simulink model "SECURE_Russia_EU_Ukraine_gas_pipeline"  (Simulink 10.3)
settings: Solver=ode45  StartTime=0.0  StopTime=100  RelTol=1e-3  EnableMultiTasking=on
undefined symbols (not defined in the file): Tab, Tba, Tca, Tcb
settings Model: Creator=Luan Nguyen  LastModifiedBy=fmendoz2  MultithreadedSim=on
settings DataIOCC: LimitDataPoints=on
settings DebuggingCC: IgnoredZcDiagnostic=none  MultiTaskDSMMsg=warning  MultiTaskCondExecSysMsg=none  FcnCallInpInsideContextMsg=error
settings GRTTargetCC: CombineOutputUpdateFcns=on  GRTInterface=off
settings ConfigComp: CovSFcnEnable=off

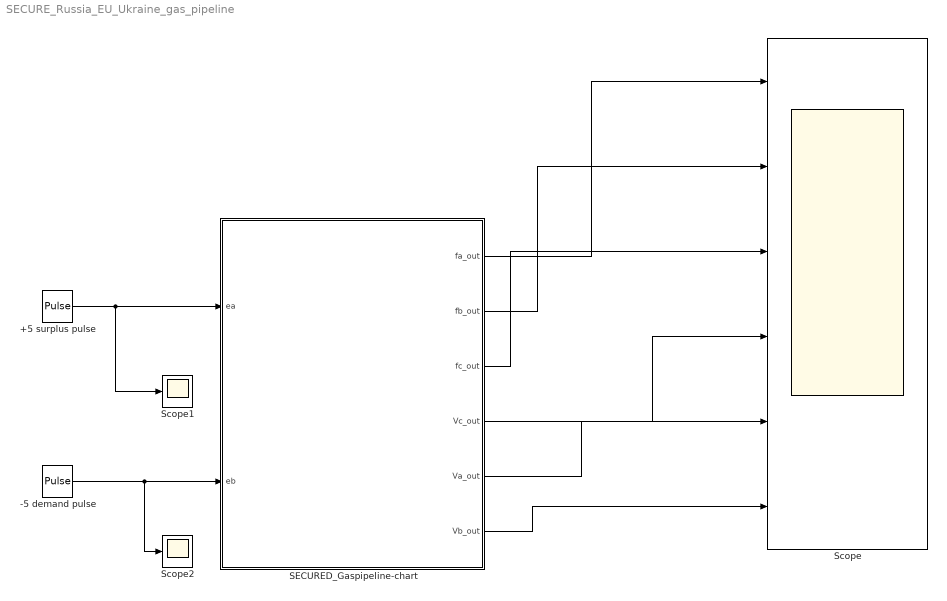
== system SECURE_Russia_EU_Ukraine_gas_pipeline ==
  +5 surplus pulse : DiscretePulseGenerator  PulseType=Time based  Amplitude=5  Period=10
  -5 demand pulse : DiscretePulseGenerator  PulseType=Time based  Amplitude=-5  Period=10
  SECURED_Gaspipeline-chart : Stateflow chart  TreatAsAtomicUnit=on
  Scope : Scope  NumInputPorts=6
  Scope1 : Scope
  Scope2 : Scope
  wires:
  SECURED_Gaspipeline-chart/1(fa_out) -> Scope/1
  SECURED_Gaspipeline-chart/2(fb_out) -> Scope/2
  SECURED_Gaspipeline-chart/3(fc_out) -> Scope/3
  SECURED_Gaspipeline-chart/4(Vc_out) -> Scope/4
  SECURED_Gaspipeline-chart/5(Va_out) -> Scope/5
  SECURED_Gaspipeline-chart/6(Vb_out) -> Scope/6
  +5 surplus pulse/1 -> Scope1/1, SECURED_Gaspipeline-chart/1(ea)
  -5 demand pulse/1 -> Scope2/1, SECURED_Gaspipeline-chart/2(eb)

== stateflow chart SECURED_Gaspipeline-chart ==
  settings: updateMethod=CONTINUOUS
  state SECURE_B_controller_Ukraine [parallel]
    settings: executionOrder=1
    state ModeB1
      du:
      zb_dot = 1;
    state ModeB3
      du:
      zb_dot = 1;
    state ModeB2
      du:
      zb_dot = 1;
    (default) -> ModeB1 : {fb = 5; fc = 10; fa = 5; zb = 0; tmpB = 0;}
    ModeB1 -> ModeB2 [order 1] : [eb >= 0]{tmpB = eb;zb = 0;}
    ModeB2 -> ModeB1 : [zb >= Tcb]
        | {fb = fb+tmpB; zb = 0;}
    ModeB3 -> ModeB1 : [zb >= 1]
        | {fb = fb+ tmpB;zb = 0;}
    ModeB1 -> ModeB3 [order 2] : [eb <= 0 ]
        | {tmpB = eb;zb = 0;}
  state SECURE_A_controller_EU [parallel]
    settings: executionOrder=2
    state ModeA5
      du:
      za_dot = 1;
    state ModeA2
      du:
      za_dot = 1;
    state ModeA1
      du:
      za_dot = 1;
    (default) -> ModeA1 : {za = 0;tmpA = 0;}
    ModeA1 -> ModeA2 [order 1] : [ea > 0]{tmpA = ea;za = 0;}
    ModeA2 -> ModeA1 : [za >= Tca]
        | {fa = fa+tmpA; za = 0;}
    ModeA5 -> ModeA1 : [za >= 1]
        | {fa = fa+ tmpA;za = 0;}
    ModeA1 -> ModeA5 [order 2] : [ea <= 0 ]
        | {tmpA = ea;za = 0}
  state SECURE_C_controller_Russia [parallel]
    settings: executionOrder=3
    state C2
      du:
      zc_dot = 1;
    state C1
      du:
      zc_dot = 1;
    (default) -> C1 : {zc = 0; tmpC = 0;}
    C2 -> C1 : [zc >=1]
        | {fc = fc+tmpC; zc = 0;}
    C1 -> C2 : [ea +eb >0 || ea + eb <0]
        | {tmpC = ea+eb;}
  state PlantModel [parallel]
    settings: executionOrder=4
    state Plant
      du:
      Va_dot = fa; Va_out = Va; fa_dot = 0; fa_out = fa;
      Vb_dot = fb; Vb_out = Vb; fb_dot = 0; fb_out = fb;
      Vc_dot = fc; Vc_out = Vc; fc_dot = 0; fc_out = fc;
  data: za local double; zb local double; fa local double; fa_out output double; ea input double; fb local double; fb_out output double; fc local double; fc_out output double; Va local double; Vb local double; Vc local double; Vc_out output double; Va_out output double; Vb_out output double; Tba parameter double; Tca parameter double; Tcb parameter double; eb input double; Tab parameter double; zc local double; tmpA local double; tmpB local double; tmpC local double
  data za settings: updateMethod=SF_CONTINUOUS_TIME_DATA
  data zb settings: updateMethod=SF_CONTINUOUS_TIME_DATA
  data fa settings: updateMethod=SF_CONTINUOUS_TIME_DATA
  data fb settings: updateMethod=SF_CONTINUOUS_TIME_DATA
  data fc settings: updateMethod=SF_CONTINUOUS_TIME_DATA
  data Va settings: updateMethod=SF_CONTINUOUS_TIME_DATA
  data Vb settings: updateMethod=SF_CONTINUOUS_TIME_DATA
  data Vc settings: updateMethod=SF_CONTINUOUS_TIME_DATA
  data zc settings: updateMethod=SF_CONTINUOUS_TIME_DATA
